simulink model "MPC_design"  (R2018b)
settings: Solver=VariableStepAuto  StartTime=0.0  StopTime=10.0  RelTol=1e-3
values from neighbouring files (symbols this model uses):
  D = D_heel + D_h + D_yaw + D_k    [nonLinearStateSpace.m]
libraries: mpclib x1
(part 1 of 2)
settings Model: Creator=bruce  LastModifiedBy=bruce

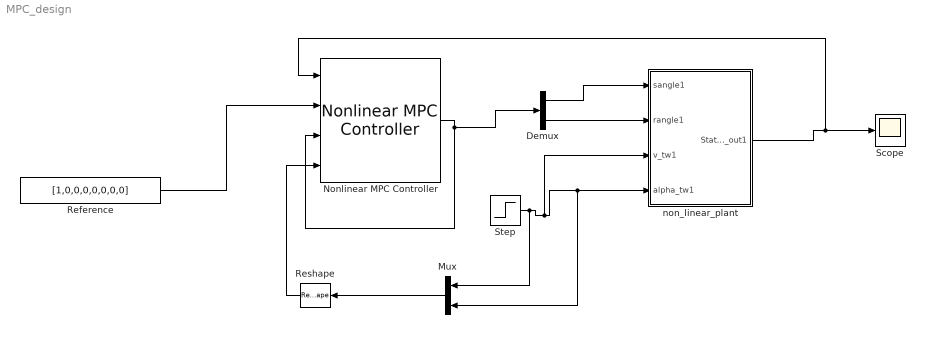
== system MPC_design ==
  Demux : Demux  Outputs=2
  Mux : Mux  Inputs=2
  Nonlinear MPC Controller : mpclib/Nonlinear MPC Controller  SCDEnableBlockLinearizationSpecification=on  nlmpcobj=nlobj  UseObjectTs=on  md_enabled=on  param_enabled=off  cost_enabled=off  mvseq_enabled=off  stateseq_enabled=off  ovseq_enabled=off  slack_enabled=off  status_enabled=off  ov_min=off  ov_max=off  mv_min=off  mv_max=off  mvrate_min=off  mvrate_max=off  state_min=off  state_max=off  ov_weight=off  mv_weight=off  mvrate_weight=off  ecr_weight=off  mvtarget_enabled=off  nlp_initialize=off
      settings: SourceProductName=Model Predictive Control Toolbox
  Reference : Constant  Value=[1,0,0,0,0,0,0,0]  VectorParams1D=off
  Reshape : Reshape  OutputDimensionality=Row vector (2-D)
  Scope : Scope
  Step : Step  Time=0  SampleTime=0
  non_linear_plant : Subsystem
  wires:
  Nonlinear MPC Controller/1 -> Demux/1, Nonlinear MPC Controller/3
  Demux/1 -> non_linear_plant/1(sangle1)
  Demux/2 -> non_linear_plant/2(rangle1)
  Step/1 -> Mux/1, non_linear_plant/3(v_tw1), Mux/2, non_linear_plant/4(alpha_tw1)
  non_linear_plant/1(States_out1) -> Nonlinear MPC Controller/1, Scope/1
  Mux/1 -> Reshape/1
  Reference/1 -> Nonlinear MPC Controller/2
  Reshape/1 -> Nonlinear MPC Controller/4

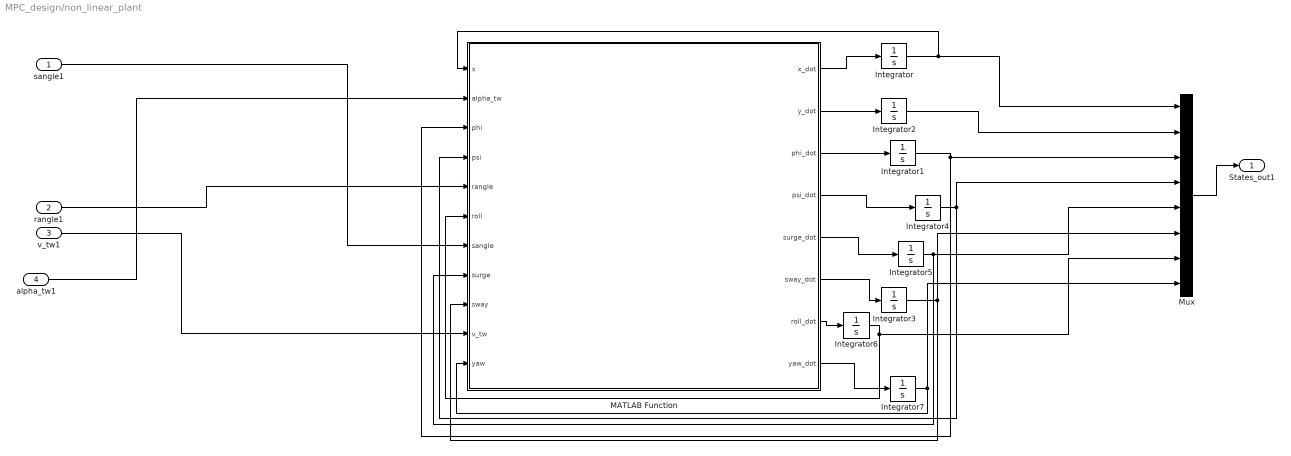
== system MPC_design/non_linear_plant ==
  sangle1 : Inport
  rangle1 : Inport  Port=2
  v_tw1 : Inport  Port=3
  alpha_tw1 : Inport  Port=4
  Integrator{,1..2,4..7} (7 alike) : Integrator  InitialCondition=0.00000001
  Integrator3 : Integrator  InitialCondition=10^(-60)
  MATLAB Function : MATLAB Function  TreatAsAtomicUnit=on
  Mux : Mux  Inputs=8
  States_out1 : Outport
  wires:
  alpha_tw1/1 -> MATLAB Function/2(alpha_tw)
  Integrator6/1 -> Mux/7, MATLAB Function/6(roll)
  v_tw1/1 -> MATLAB Function/10(v_tw)
  Integrator3/1 -> Mux/6, MATLAB Function/9(sway)
  Integrator/1 -> MATLAB Function/1(x), Mux/1
  Integrator1/1 -> MATLAB Function/3(phi), Mux/3
  Mux/1 -> States_out1/1
  MATLAB Function/6(sway_dot) -> Integrator3/1
  Integrator7/1 -> MATLAB Function/11(yaw), Mux/8
  Integrator4/1 -> MATLAB Function/4(psi), Mux/4
  MATLAB Function/2(y_dot) -> Integrator2/1
  MATLAB Function/1(x_dot) -> Integrator/1
  MATLAB Function/3(phi_dot) -> Integrator1/1
  MATLAB Function/7(roll_dot) -> Integrator6/1
  MATLAB Function/5(surge_dot) -> Integrator5/1
  MATLAB Function/8(yaw_dot) -> Integrator7/1
  Integrator5/1 -> Mux/5, MATLAB Function/8(surge)
  MATLAB Function/4(psi_dot) -> Integrator4/1
  rangle1/1 -> MATLAB Function/5(rangle)
  sangle1/1 -> MATLAB Function/7(sangle)
  Integrator2/1 -> Mux/2
